simulink model "questao5_prova3"  (Simulink 7.9)
settings: Solver=ode45  StartTime=0.0  StopTime=40.0  RelTol=1e-3
settings Model: Creator=Danilo  LastModifiedBy=Danilo

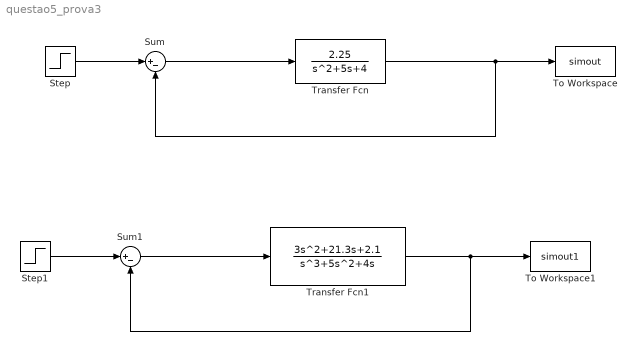
== system questao5_prova3 ==
  Step : Step  Time=0  SampleTime=0
  Step1 : Step  Time=0  SampleTime=0
  Sum : Sum  Inputs=|+-
  Sum1 : Sum  Inputs=|+-
  To Workspace : ToWorkspace  VariableName=simout  SampleTime=-1
  To Workspace1 : ToWorkspace  VariableName=simout1  SampleTime=-1
  Transfer Fcn : TransferFcn  Numerator=[2.25]  Denominator=[1 5 4]
  Transfer Fcn1 : TransferFcn  Numerator=[3 21.3 2.1]  Denominator=[1 5 4 0]
  wires:
  Step/1 -> Sum/1
  Sum/1 -> Transfer Fcn/1
  Transfer Fcn/1 -> To Workspace/1, Sum/2
  Step1/1 -> Sum1/1
  Transfer Fcn1/1 -> To Workspace1/1, Sum1/2
  Sum1/1 -> Transfer Fcn1/1
